simulink model "cp_statefeedback_final"  (R2014a)
settings: Solver=ode45  StartTime=0.0  StopTime=50  RelTol=1e-3
values from neighbouring files (symbols this model uses):
  A = [ 0 -(M+m)*g/(M*l) kf/(M*l) 0 ; 1 0 0 0 ; 0 m*g/M -kf/M 0 ; 0 0 1 0 ]    [CPscript_friction.m]    (also in fixedptscript_R0.m = [ 0 -(M+m)*g/(M*l) 0 0 ; 1 0 0 0 ; 0 m*g/M 0 0 ; 0 0 1 0 ])
  B = [-1/(M*l); 0; 1/M ;0 ]    [CPscript_friction.m]    (also in fixedptscript_R0.m)
  C = eye(4)    [CPscript_friction.m]    (also in fixedptscript_R0.m)
  D = [0; 0; 0; 0]    [CPscript_friction.m]    (also in fixedptscript_R0.m)
  F_0 = 1    [CPscript_friction.m]    (also in fixedptscript_R0.m)
  F_i = 22.0532    [CPscript_friction.m]    (also in fixedptscript_R0.m)
  g = 9.80665    [CPscript_friction.m]    (also in fixedptscript_R0.m)
  KD = [(F_i/omega_i) (F_i*alpha_0/alpha_i) F_i/vel_i  F_i/x_i].*(kt_dg)    [CPscript_friction.m]    (also in fixedptscript_R0.m)
  kd_i = [omega_i 0 0 0 ; 0 (alpha_i/alpha_0) 0 0 ; 0 0 vel_i 0 ; 0 0 0 (x_i/x_0)]    [CPscript_friction.m]    (also in fixedptscript_R0.m)
  ki = -k1(5)    [CPscript_friction.m]    (also in fixedptscript_R0.m)
  ki_d = -kt_d(5)*Ts    [CPscript_friction.m]    (also in fixedptscript_R0.m)
  KI_D = (x_0/x_i)* ki_d *(F_i/F_0)    [CPscript_friction.m]    (also in fixedptscript_R0.m)
  KP_D = (x_0/x_i)* p *(F_i/F_0)    [CPscript_friction.m]    (also in fixedptscript_R0.m)
  kt_dg = kt_d(1:4)-p*Ctk    [CPscript_friction.m]    (also in fixedptscript_R0.m)
  kt_pi = k1(1:4)-p*Ctk    [CPscript_friction.m]    (also in fixedptscript_R0.m)
  l = 0.285    [CPscript_friction.m]    (also in fixedptscript_R0.m)
  LIMIT_INT = round(limit * 2^KI_SHIFT)    [CPscript_friction.m]    (also in fixedptscript_R0.m)
  M = 4.676    [CPscript_friction.m]    (also in fixedptscript_R0.m)
  m = 0.098    [CPscript_friction.m]    (also in fixedptscript_R0.m)
  p = 1/([0 0 0 1]*(((B*k)-A)^-1)*B)    [CPscript_friction.m]    (also in fixedptscript_R0.m)
  Ts = 10e-3    (= 0.01)    [CPscript_friction.m]    (also in fixedptscript_R0.m)
  x_0 = 1    [CPscript_friction.m]    (also in fixedptscript_R0.m)
  x_i = 28619    [CPscript_friction.m]    (also in fixedptscript_R0.m)
settings Model: Creator=Jimit Kavathia  LastModifiedBy=iae
settings OptimizationCC: BlockReduction=off  BooleanDataType=off  SimCompilerOptimization=off
settings DebuggingCC: SaveWithParameterizedLinksMsg=none  UnderspecifiedInitializationDetection=Classic  SignalResolutionControl=TryResolveAllWithWarning  SolverPrmCheckMsg=none  FcnCallInpInsideContextMsg=error  FrameProcessingCompatibilityMsg=error  SFExecutionAtInitializationDiag=none
settings HardwareCC: ProdBitPerSizeT=32  ProdBitPerPtrDiffT=32  TargetUnknown=on
settings RTWCC: RTWCompilerOptimization=off
settings CodeAppCC: StateflowObjectComments=on
settings ConfigComp: CovMetricSettings=dw  CovHtmlReporting=on  CovSaveCumulativeToWorkspaceVar=on  CovSaveSingleToWorkspaceVar=on  CovExternalEMLEnable=off

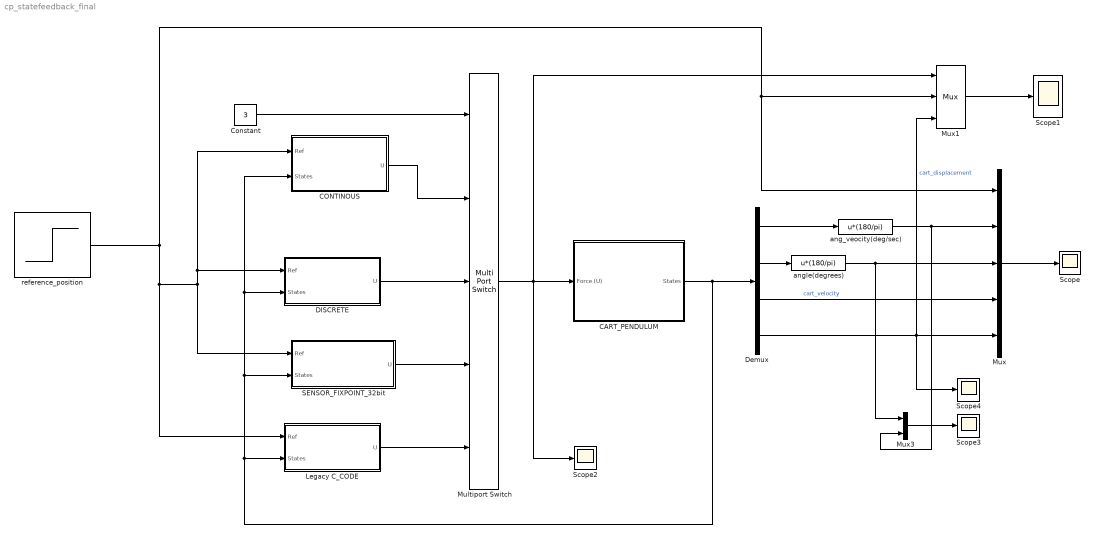
== system cp_statefeedback_final ==
  CART_PENDULUM : Subsystem
  CONTINOUS : Subsystem
  Constant : Constant  Value=3
  DISCRETE : Subsystem
  Demux : Demux
  Legacy C_CODE : Subsystem
  Multiport Switch : MultiPortSwitch  Inputs=4
  Mux : Mux  Inputs=5
  Mux1 : Mux  Inputs=3
  Mux3 : Mux  Inputs=2
  SENSOR_FIXPOINT_32bit : Subsystem
  Scope{,1..4} (5 alike) : Scope
  ang_veocity(deg/sec) : Fcn  Expr=u*(180/pi)
  angle(degrees) : Fcn  Expr=u*(180/pi)
  reference_position : Step  SampleTime=0
  wires:
  CONTINOUS/1(U) -> Multiport Switch/2
  DISCRETE/1(U) -> Multiport Switch/3
  Constant/1 -> Multiport Switch/1
  CART_PENDULUM/1(States) -> Demux/1, CONTINOUS/2(States), DISCRETE/2(States), SENSOR_FIXPOINT_32bit/2(States), Legacy C_CODE/2(States)
  Demux/3 -> Mux/4  "cart_velocity"
  Demux/4 -> Scope4/1, Mux1/3, Mux/5  "cart_displacement"
  angle(degrees)/1 -> Mux3/1, Mux/3
  Demux/2 -> angle(degrees)/1
  ang_veocity(deg/sec)/1 -> Mux3/2, Mux/2
  Demux/1 -> ang_veocity(deg/sec)/1
  Mux/1 -> Scope/1
  Mux1/1 -> Scope1/1
  Multiport Switch/1 -> Mux1/1, CART_PENDULUM/1(Force (U)), Scope2/1
  Mux3/1 -> Scope3/1
  reference_position/1 -> Mux1/2, Mux/1, Legacy C_CODE/1(Ref), SENSOR_FIXPOINT_32bit/1(Ref), CONTINOUS/1(Ref), DISCRETE/1(Ref)
  SENSOR_FIXPOINT_32bit/1(U) -> Multiport Switch/4
  Legacy C_CODE/1(U) -> Multiport Switch/5

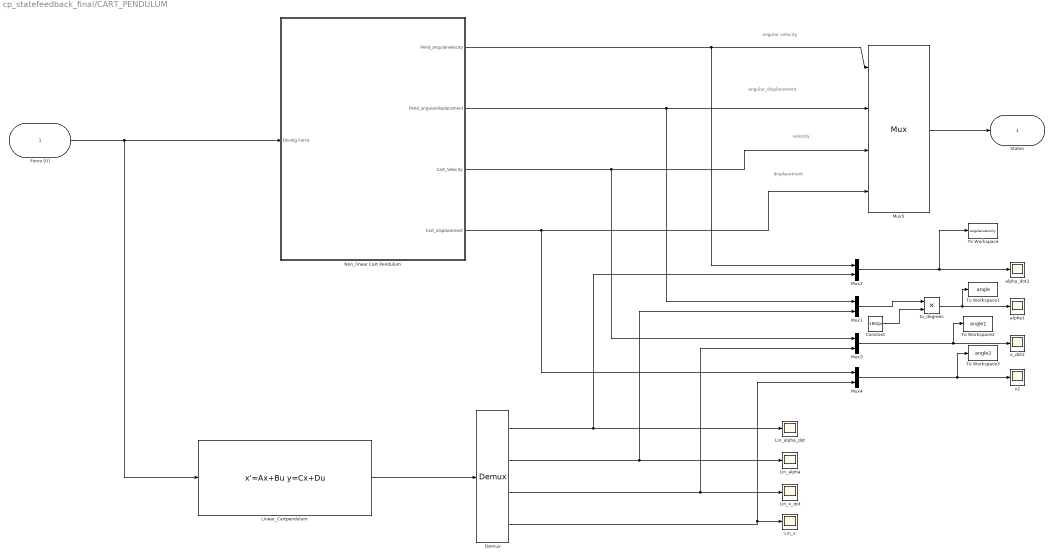
== system cp_statefeedback_final/CART_PENDULUM ==
  note: angular velocity
  note: angular_displacement
  note: displacement
  note: velocity
  Force (U) : Inport
  Constant : Constant  Value=180/pi
  Demux : Demux
  Lin_alpha : Scope
  Lin_alpha_dot : Scope
  Lin_x : Scope
  Lin_x_dot : Scope
  Linear_Cartpendulum : StateSpace  A=A  B=B  C=C  D=D
  Mux{1..4} (4 alike) : Mux  Inputs=2
  Mux5 : Mux
      settings: DisplayOption=signals
  Non_linear Cart Pendulum : Subsystem
  To Workspace : ToWorkspace  VariableName=angularvelocity  SaveFormat=Timeseries  SampleTime=-1
  To Workspace1 : ToWorkspace  VariableName=angle  SaveFormat=Timeseries  SampleTime=-1
  To Workspace2 : ToWorkspace  VariableName=angle1  SaveFormat=Timeseries  SampleTime=-1
  To Workspace3 : ToWorkspace  VariableName=angle2  SaveFormat=Timeseries  SampleTime=-1
  alpha1 : Scope
  alpha_dot2 : Scope
  to_degrees : Product  Inputs=**
  x2 : Scope
  x_dot2 : Scope
  States : Outport
  wires:
  Non_linear Cart Pendulum/2("                   Pend_angulardisplacement") -> Mux1/1, Mux5/2
  Non_linear Cart Pendulum/3(Cart_Velocity) -> Mux3/1, Mux5/3
  Mux5/1 -> States/1
  Mux1/1 -> to_degrees/1
  Non_linear Cart Pendulum/1("                   Pend_angularvelocity") -> Mux2/1, Mux5/1
  Demux/1 -> Mux2/2, Lin_alpha_dot/1
  Demux/4 -> Mux4/2, Lin_x/1
  to_degrees/1 -> To Workspace1/1, alpha1/1
  Mux2/1 -> To Workspace/1, alpha_dot2/1
  Non_linear Cart Pendulum/4(Cart_displacement) -> Mux4/1, Mux5/4
  Constant/1 -> to_degrees/2
  Mux3/1 -> To Workspace2/1, x_dot2/1
  Linear_Cartpendulum/1 -> Demux/1
  Mux4/1 -> To Workspace3/1, x2/1
  Demux/2 -> Mux1/2, Lin_alpha/1
  Demux/3 -> Mux3/2, Lin_x_dot/1
  Force (U)/1 -> Linear_Cartpendulum/1, Non_linear Cart Pendulum/1(Driving Force)

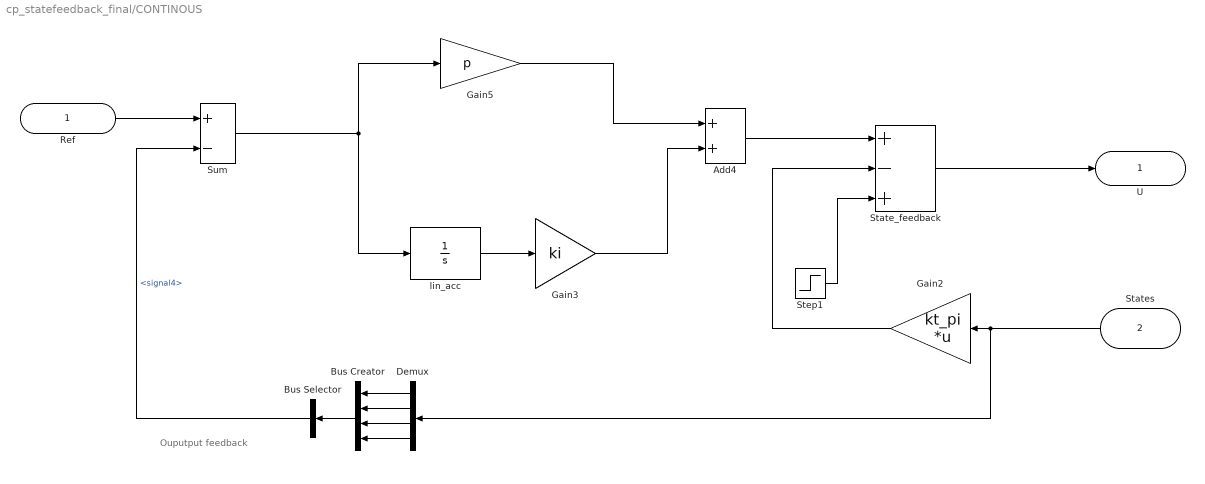
== system cp_statefeedback_final/CONTINOUS ==
  note: Ouputput feedback
  Ref : Inport
  States : Inport  Port=2
  Add4 : Sum
  Bus Creator : BusCreator
  Bus Selector : BusSelector  OutputSignals=signal4
  Demux : Demux
  Gain2 : Gain  Gain=kt_pi  Multiplication=Matrix(K*u) (u vector)
  Gain3 : Gain  Gain=ki
  Gain5 : Gain  Gain=p
  State_feedback : Sum  Inputs=+-+
  Step1 : Step  Time=10  After=0  SampleTime=0
  Sum : Sum  Inputs=+-
  lin_acc : Integrator
  U : Outport
  wires:
  State_feedback/1 -> U/1
  Gain5/1 -> Add4/1
  Add4/1 -> State_feedback/1
  Gain3/1 -> Add4/2
  Sum/1 -> lin_acc/1, Gain5/1
  Step1/1 -> State_feedback/3
  lin_acc/1 -> Gain3/1
  States/1 -> Demux/1, Gain2/1
  Ref/1 -> Sum/1
  Bus Selector/1 -> Sum/2  "<signal4>"
  Gain2/1 -> State_feedback/2
  Demux/1 -> Bus Creator/1
  Demux/2 -> Bus Creator/2
  Demux/3 -> Bus Creator/3
  Demux/4 -> Bus Creator/4
  Bus Creator/1 -> Bus Selector/1

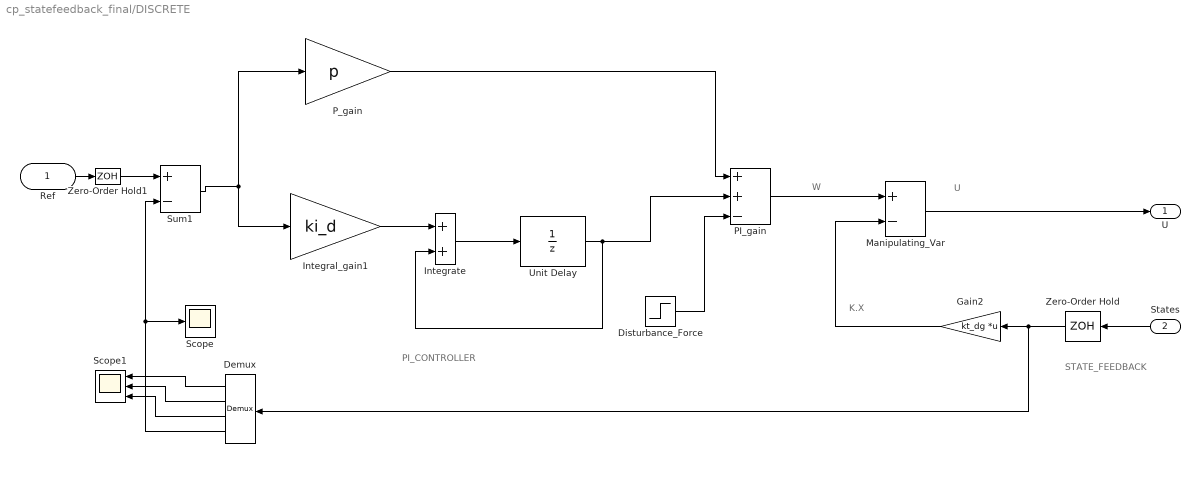
== system cp_statefeedback_final/DISCRETE ==
  note: PI_CONTROLLER
  note: W
  note: K.X
  note: U
  note: STATE_FEEDBACK
  Ref : Inport
  States : Inport  Port=2
  Demux : Demux
  Disturbance_Force : Step  Time=0  After=0  SampleTime=Ts
  Gain2 : Gain  Gain=kt_dg  Multiplication=Matrix(K*u) (u vector)
  Integral_gain1 : Gain  Gain=ki_d
  Integrate : Sum
  Manipulating_Var : Sum  Inputs=+-
  PI_gain : Sum  Inputs=++-
  P_gain : Gain  Gain=p
  Scope : Scope
  Scope1 : Scope  NumInputPorts=3
      settings: YMin=-5~-5~-5  YMax=5~5~5
  Sum1 : Sum  Inputs=+-
  Unit Delay : UnitDelay  SampleTime=Ts
  Zero-Order Hold : ZeroOrderHold  SampleTime=Ts
  Zero-Order Hold1 : ZeroOrderHold  SampleTime=Ts
  U : Outport
  wires:
  Manipulating_Var/1 -> U/1
  States/1 -> Zero-Order Hold/1
  PI_gain/1 -> Manipulating_Var/1
  P_gain/1 -> PI_gain/1
  Integrate/1 -> Unit Delay/1
  Unit Delay/1 -> Integrate/2, PI_gain/2
  Sum1/1 -> P_gain/1, Integral_gain1/1
  Disturbance_Force/1 -> PI_gain/3
  Ref/1 -> Zero-Order Hold1/1
  Demux/4 -> Scope/1, Sum1/2
  Gain2/1 -> Manipulating_Var/2
  Zero-Order Hold/1 -> Demux/1, Gain2/1
  Integral_gain1/1 -> Integrate/1
  Zero-Order Hold1/1 -> Sum1/1
  Demux/1 -> Scope1/1
  Demux/2 -> Scope1/2
  Demux/3 -> Scope1/3

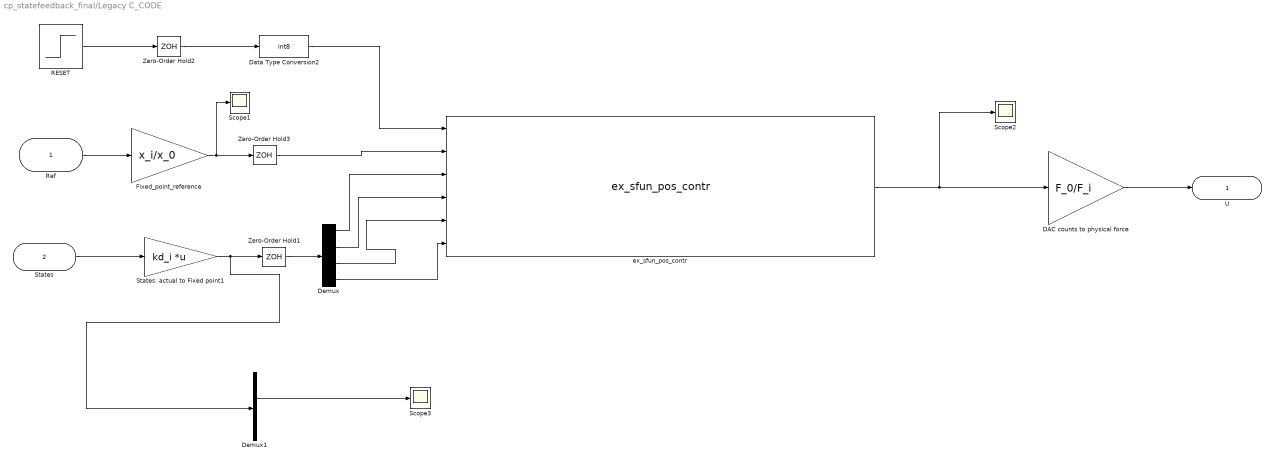
== system cp_statefeedback_final/Legacy C_CODE ==
  Ref : Inport
  States : Inport  Port=2
  " DAC counts to physical force" : Gain  Gain=F_0/F_i  ParamDataTypeStr=double  OutDataTypeStr=double
  Data Type Conversion2 : DataTypeConversion  OutDataTypeStr=int8
  Demux : Demux
  Demux1 : Demux
  Fixed_point_reference : Gain  Gain=x_i/x_0  OutDataTypeStr=int16
  RESET : Step  Time=3*Ts  Before=1  After=0  SampleTime=Ts
  Scope1 : Scope
  Scope2 : Scope
  Scope3 : Scope
  States: actual to Fixed point1 : Gain  Gain=kd_i  Multiplication=Matrix(K*u) (u vector)  OutDataTypeStr=int16
  Zero-Order Hold1 : ZeroOrderHold  SampleTime=Ts
  Zero-Order Hold2 : ZeroOrderHold  SampleTime=Ts
  Zero-Order Hold3 : ZeroOrderHold  SampleTime=Ts
  ex_sfun_pos_contr : S-Function  FunctionName=ex_sfun_pos_contr  EnableBusSupport=off  mask(Legacy Function){SFunctionSpec=int16 y1 = pos_contr(int8 u1, int16 u2, int16 u3, int16 u4, int16 u5, int16 u6), ShowSpec=on}
      mask prompts: ShowSpec "Display function specification"
      mask help:
      | This block allows you to call the legacy functions specified by the following Legacy Code Tool definition:
      | def.SFunctionName = 'ex_sfun_pos_contr';
      | def.OutputFcnSpec = 'int16 y1 = pos_contr(int8 u1, int16 u2, int16 u3, int16 u4, int16 u5, int16 u6)';
      | def.HeaderFiles = {'stfbk_control.h', 'xil_types.h', 'pi_control.h'};
      | def.SourceFiles = {'pos_contr.c', 'stfbk_control.c', 'pi_control.c'};
      mask Help: <p>This block was generated automatically by the Legacy Code Tool. For detailed help on this tool, call<a href="matlab:legacy_code('help')"> legacy_code('help')</a>.</p>
      mask Callback ShowSpec:
      | if strcmp(get_param(gcbh, 'ShowSpec'), 'on')
      |   set_param(gcbh, 'MaskDisplay', sprintf('fprintf(''%s'');', get_param(gcbh, 'SFunctionSpec')));
      | else
      |   set_param(gcbh, 'MaskDisplay', sprintf('fprintf(''%s'');', get_param(gcbh, 'FunctionName')));
      | end
      mask Display: fprintf('int16 y1 = pos_contr(int8 u1, int16 u2, int16 u3, int16 u4, int16 u5, int16 u6)');
  U : Outport
  wires:
  Zero-Order Hold1/1 -> Demux/1
  RESET/1 -> Zero-Order Hold2/1
  Zero-Order Hold2/1 -> Data Type Conversion2/1
  Data Type Conversion2/1 -> ex_sfun_pos_contr/1
  Fixed_point_reference/1 -> Scope1/1, Zero-Order Hold3/1
  Ref/1 -> Fixed_point_reference/1
  Zero-Order Hold3/1 -> ex_sfun_pos_contr/2
  Demux/1 -> ex_sfun_pos_contr/3
  Demux/2 -> ex_sfun_pos_contr/4
  Demux/3 -> ex_sfun_pos_contr/5
  Demux/4 -> ex_sfun_pos_contr/6
  ex_sfun_pos_contr/1 -> " DAC counts to physical force"/1, Scope2/1
  States/1 -> States: actual to Fixed point1/1
  " DAC counts to physical force"/1 -> U/1
  Demux1/2 -> Scope3/1
  States: actual to Fixed point1/1 -> Demux1/1, Zero-Order Hold1/1

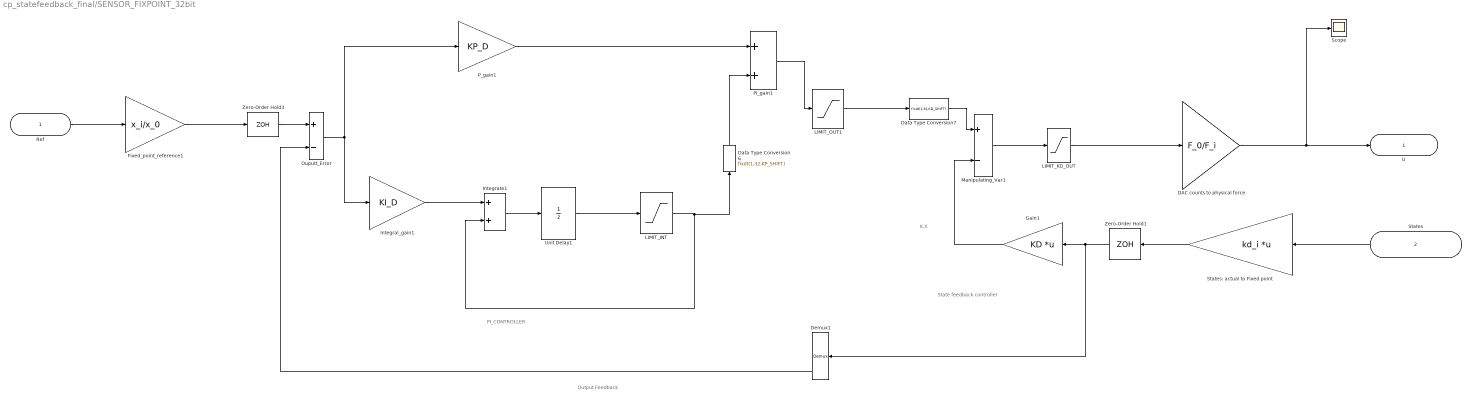
== system cp_statefeedback_final/SENSOR_FIXPOINT_32bit ==
  note: K.X
  note: PI_CONTROLLER
  note: Output Feedback
  note: State feedback controller
  Ref : Inport
  States : Inport  Port=2
  " DAC counts to physical force" : Gain  Gain=F_0/F_i  ParamDataTypeStr=double  OutDataTypeStr=double
  Data Type Conversion6 : DataTypeConversion  OutDataTypeStr=fixdt(1,32,KP_SHIFT)
  Data Type Conversion7 : DataTypeConversion  OutDataTypeStr=fixdt(1,32,KD_SHIFT)
  Demux1 : Demux
  Fixed_point_reference1 : Gain  Gain=x_i/x_0  OutDataTypeStr=int16
  Gain1 : Gain  Gain=KD  Multiplication=Matrix(K*u) (u vector)  ParamDataTypeStr=fixdt(1,16,KD_SHIFT)
  Integral_gain1 : Gain  Gain=KI_D  ParamDataTypeStr=fixdt(1,16,KI_SHIFT)
  Integrate1 : Sum
  LIMIT_INT : Saturate  UpperLimit=LIMIT_INT  LowerLimit=-LIMIT_INT
  LIMIT_KD_OUT : Saturate  UpperLimit=1048064  LowerLimit=-1048064
  LIMIT_OUT1 : Saturate  UpperLimit=16384  LowerLimit=-16384
  Manipulating_Var1 : Sum  Inputs=+-
  Ouputt_Error : Sum  Inputs=+-
  PI_gain1 : Sum
  P_gain1 : Gain  Gain=KP_D  ParamDataTypeStr=fixdt(1,16,KP_SHIFT)
  Scope : Scope
  States: actual to Fixed point : Gain  Gain=kd_i  Multiplication=Matrix(K*u) (u vector)  OutDataTypeStr=int16
  Unit Delay1 : UnitDelay  SampleTime=Ts
  Zero-Order Hold1 : ZeroOrderHold  SampleTime=Ts
  Zero-Order Hold3 : ZeroOrderHold  SampleTime=Ts
  U : Outport
  wires:
  PI_gain1/1 -> LIMIT_OUT1/1
  States/1 -> States: actual to Fixed point/1
  LIMIT_INT/1 -> Data Type Conversion6/1, Integrate1/2
  Zero-Order Hold3/1 -> Ouputt_Error/1
  States: actual to Fixed point/1 -> Zero-Order Hold1/1
  " DAC counts to physical force"/1 -> Scope/1, U/1
  Data Type Conversion7/1 -> Manipulating_Var1/1
  Unit Delay1/1 -> LIMIT_INT/1
  Ouputt_Error/1 -> P_gain1/1, Integral_gain1/1
  Demux1/4 -> Ouputt_Error/2
  Ref/1 -> Fixed_point_reference1/1
  Integrate1/1 -> Unit Delay1/1
  P_gain1/1 -> PI_gain1/1
  Manipulating_Var1/1 -> LIMIT_KD_OUT/1
  Zero-Order Hold1/1 -> Gain1/1, Demux1/1
  LIMIT_OUT1/1 -> Data Type Conversion7/1
  Fixed_point_reference1/1 -> Zero-Order Hold3/1
  Gain1/1 -> Manipulating_Var1/2
  LIMIT_KD_OUT/1 -> " DAC counts to physical force"/1
  Integral_gain1/1 -> Integrate1/1
  Data Type Conversion6/1 -> PI_gain1/2

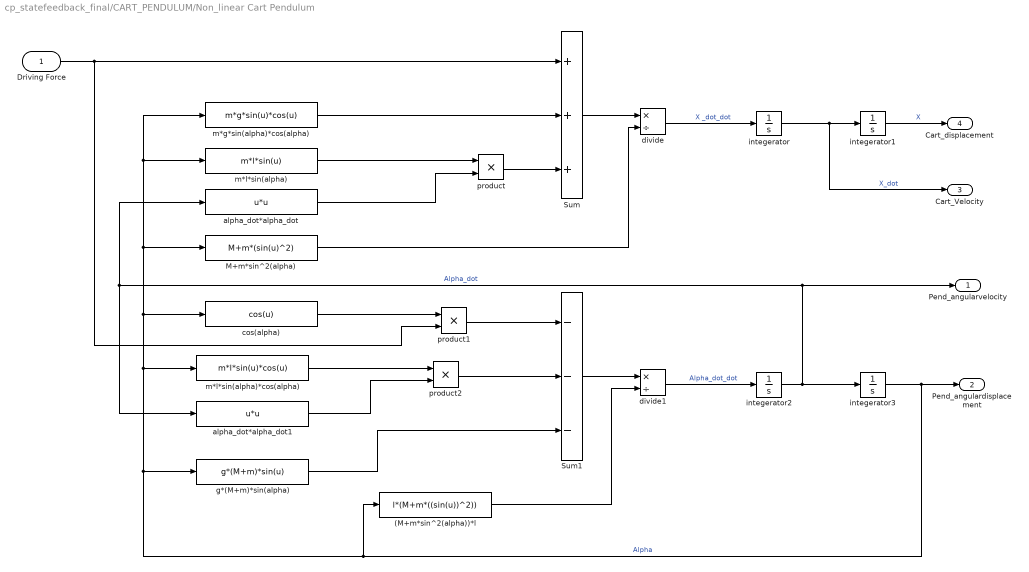
== system cp_statefeedback_final/CART_PENDULUM/Non_linear Cart Pendulum ==
  Driving Force : Inport
  (M+m*sin^2(alpha))*l : Fcn  Expr=l*(M+m*((sin(u))^2))
  M+m*sin^2(alpha) : Fcn  Expr=M+m*(sin(u)^2)
  Sum : Sum  Inputs=+++
  Sum1 : Sum  Inputs=---
  alpha_dot*alpha_dot : Fcn  Expr=u*u
  alpha_dot*alpha_dot1 : Fcn  Expr=u*u
  cos(alpha) : Fcn  Expr=cos(u)
  divide : Product  Inputs=*/
  divide1 : Product  Inputs=*/  OutDataTypeStr=double
  g*(M+m)*sin(alpha) : Fcn  Expr=g*(M+m)*sin(u)
  integerator{,1..3} (4 alike) : Integrator
  m*g*sin(alpha)*cos(alpha) : Fcn  Expr=m*g*sin(u)*cos(u)
  m*l*sin(alpha) : Fcn  Expr=m*l*sin(u)
  m*l*sin(alpha)*cos(alpha) : Fcn  Expr=m*l*sin(u)*cos(u)
  product : Product
  product1 : Product  OutDataTypeStr=double
  product2 : Product
  "                   Pend_angularvelocity" : Outport
  "                   Pend_angulardisplacement" : Outport  Port=2
  Cart_Velocity : Outport  Port=3
  Cart_displacement : Outport  Port=4
  wires:
  product1/1 -> Sum1/1
  Driving Force/1 -> Sum/1, product1/2
  divide1/1 -> integerator2/1  "Alpha_dot_dot"
  cos(alpha)/1 -> product1/1
  m*g*sin(alpha)*cos(alpha)/1 -> Sum/2
  integerator1/1 -> Cart_displacement/1  "X"
  integerator2/1 -> integerator3/1, "                   Pend_angularvelocity"/1, alpha_dot*alpha_dot1/1, alpha_dot*alpha_dot/1  "Alpha_dot"
  integerator/1 -> Cart_Velocity/1, integerator1/1  "X_dot"
  Sum/1 -> divide/1
  integerator3/1 -> "                   Pend_angulardisplacement"/1, g*(M+m)*sin(alpha)/1, m*l*sin(alpha)*cos(alpha)/1, cos(alpha)/1, M+m*sin^2(alpha)/1, m*l*sin(alpha)/1, m*g*sin(alpha)*cos(alpha)/1, (M+m*sin^2(alpha))*l/1  "Alpha"
  divide/1 -> integerator/1  "X _dot_dot"
  m*l*sin(alpha)*cos(alpha)/1 -> product2/1
  g*(M+m)*sin(alpha)/1 -> Sum1/3
  m*l*sin(alpha)/1 -> product/1
  alpha_dot*alpha_dot/1 -> product/2
  M+m*sin^2(alpha)/1 -> divide/2
  alpha_dot*alpha_dot1/1 -> product2/2
  product/1 -> Sum/3
  (M+m*sin^2(alpha))*l/1 -> divide1/2
  Sum1/1 -> divide1/1
  product2/1 -> Sum1/2
